simulink model "SP_pitch"  (R2013b)
settings: Solver=ode3  StartTime=0.0  StopTime=10  FixedStep=0.001  RelTol=1e-3
settings Model: Creator=Zhaolei  LastModifiedBy=Zhaolei

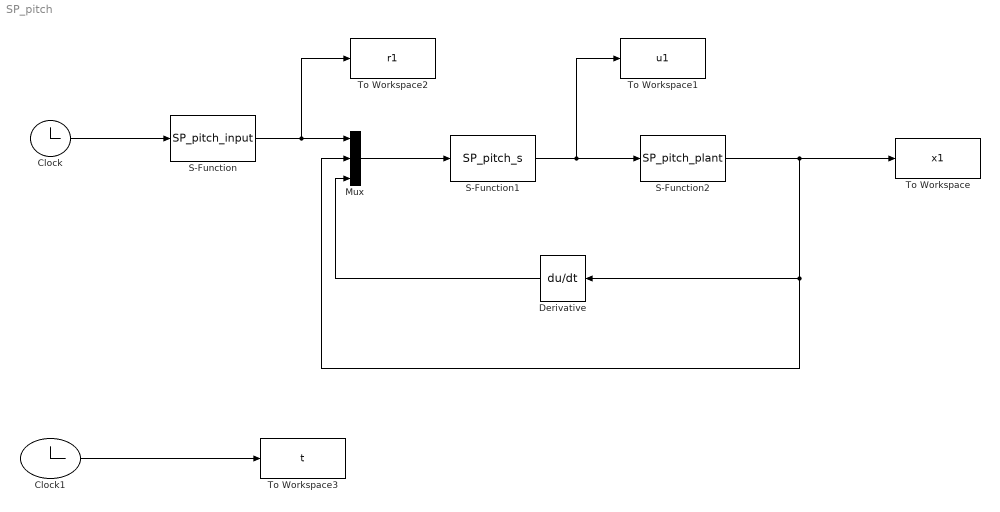
== system SP_pitch ==
  Clock : Clock
  Clock1 : Clock
  Derivative : Derivative
  Mux : Mux  Inputs=3
  S-Function : S-Function  FunctionName=SP_pitch_input  EnableBusSupport=off
  S-Function1 : S-Function  FunctionName=SP_pitch_s  EnableBusSupport=off
  S-Function2 : S-Function  FunctionName=SP_pitch_plant  EnableBusSupport=off
  To Workspace : ToWorkspace  VariableName=x1  SampleTime=-1
  To Workspace1 : ToWorkspace  VariableName=u1  SampleTime=-1
  To Workspace2 : ToWorkspace  VariableName=r1  SampleTime=-1
  To Workspace3 : ToWorkspace  VariableName=t  SampleTime=-1
  wires:
  Clock/1 -> S-Function/1
  Mux/1 -> S-Function1/1
  S-Function1/1 -> To Workspace1/1, S-Function2/1
  S-Function2/1 -> Mux/2, Derivative/1, To Workspace/1
  Derivative/1 -> Mux/3
  Clock1/1 -> To Workspace3/1
  S-Function/1 -> To Workspace2/1, Mux/1
